simulink model "Power_Forcasting_V1_UseThisOne"  (R2024a)
settings: Solver=VariableStepAuto  StartTime=0.0  StopTime=2154  RelTol=1e-3
undefined symbols (not defined in the file or in its folder): DiscIntNeverNeededParam
libraries: dspstat3 x2, slpidlib x1
settings Model: Creator=ezeki  LastModifiedBy=ezeki

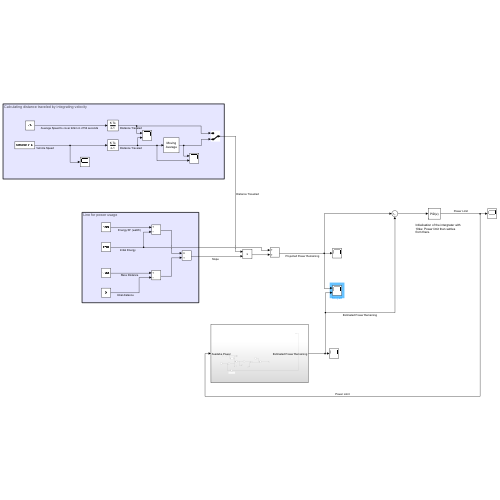
[thumbnail: Simulink's stored preview of the top-level diagram]
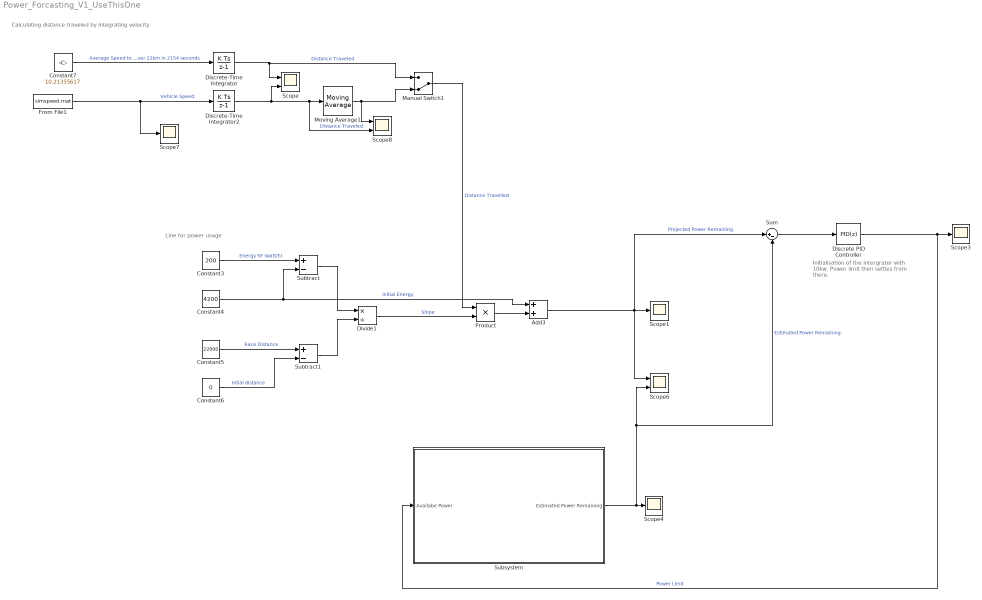
== system Power_Forcasting_V1_UseThisOne ==
  note: Calculating distance traveled by integrating velocity
  note: Line for power usage
  note: Initialisation of the intergrater with 10kw. Power limit then settles from there.
  Add3 : Sum
  Constant3 : Constant  Value=200
  Constant4 : Constant  Value=4200
  Constant5 : Constant  Value=22000
  Constant6 : Constant  Value=0
  Constant7 : Constant  Value=10.21355617
  Discrete PID Controller : slpidlib/PID Controller  Controller=PID  Form=Parallel  TimeDomain=Discrete-time  UseExternalTs=off  SampleTime=-1  IntegratorMethod=Forward Euler  FilterMethod=Forward Euler  ControllerParametersSource=internal  P=-10  I=0.001  UseKiTs=off  D=500  UseExternalDerivativeSource=off  N=0.01  UseFilter=on  TunerSelectOption=Transfer Function Based (PID Tuner App)  InitialConditionSource=internal  InitialConditionForIntegrator=10000  InitialConditionForFilter=0  DifferentiatorICPrevScaledInput=0  ExternalReset=none  TrackingMode=off  Kt=1  LimitOutput=off  SatLimitsSource=internal  UpperSaturationLimit=inf  LowerSaturationLimit=-inf  LinearizeAsGain=off  AntiWindupMode=none  Kb=1  LimitIntegrator=off  UpperIntegratorSaturationLimit=inf  LowerIntegratorSaturationLimit=-inf  POutMin=[]  POutMax=[]  IOutMin=[]  IOutMax=[]  DOutMin=[]  DOutMax=[]  NOutMin=[]  NOutMax=[]  SumOutMin=[]  SumOutMax=[]  SaturationOutMin=[]  SaturationOutMax=[]  PParamMin=[]  PParamMax=[]  IParamMin=[]  IParamMax=[]  DParamMin=[]  DParamMax=[]  NParamMin=[]  NParamMax=[]  KbParamMin=[]  KbParamMax=[]  KtParamMin=[]  KtParamMax=[]  KbOutMin=[]  KbOutMax=[]  KtOutMin=[]  KtOutMax=[]  IntegratorOutMin=[]  IntegratorOutMax=[]  FilterOutMin=[]  FilterOutMax=[]  SumI1OutMin=[]  SumI1OutMax=[]  SumI2OutMin=[]  SumI2OutMax=[]  SumI3OutMin=[]  SumI3OutMax=[]  SumI4OutMin=[]  SumI4OutMax=[]  SumDOutMin=[]  SumDOutMax=[]  DifferentiatorOutMin=[]  DifferentiatorOutMax=[]  FilterDiffOutCoefMin=[]  FilterDiffOutCoefMax=[]  ReciprocalOutMin=[]  ReciprocalOutMax=[]  SumDenOutMin=[]  SumDenOutMax=[]  SumNumOutMin=[]  SumNumOutMax=[]  DivideOutMin=[]  DivideOutMax=[]  UdiffTsProdOutMin=[]  UdiffTsProdOutMax=[]  NTsProdOutMin=[]  NTsProdOutMax=[]  UintegralTsProdOutMin=[]  UintegralTsProdOutMax=[]  UngainTsProdOutMin=[]  UngainTsProdOutMax=[]  ClampingZeroOutDataTypeStr=Inherit: Inherit via back propagation  ClampingZeroOutMin=[]  ClampingZeroOutMax=[]  FilterDenConstantOutDataTypeStr=Inherit: Inherit via back propagation  FilterDenConstantOutMin=[]  FilterDenConstantOutMax=[]  PCopyOutDataTypeStr=Inherit: Inherit via back propagation  PCopyOutMin=[]  PCopyOutMax=[]  NCopyOutDataTypeStr=Inherit: Inherit via back propagation  NCopyOutMin=[]  NCopyOutMax=[]  IntegratorContinuousStateAttributes=''  IntegratorStateMustResolveToSignalObject=off  IntegratorRTWStateStorageClass=Auto  FilterContinuousStateAttributes=''  FilterStateMustResolveToSignalObject=off  FilterRTWStateStorageClass=Auto  ParallelPVariant=InternalParameters  IdealPVariant=Disabled  IVariant=InternalParameters  DVariant=InternalParameters  IntegratorVariant=Discrete  SatVariant=Disabled  AWVariant=Passthrough  PCopyVariant=Disabled  TRVariant=Disabled  FdbkBlocksVariant=Forward  IdealPFdbkVariant=Disabled  SatFdbkVariant=Disabled  DerivativeFilterVariant=ForwardEulerFilter  NVariant=InternalParameters  NCopyVariant=Disabled  FilterICVariant=InternalICsFilter  IntegratorICVariant=InternalICs  ExternalResetVariant=Disabled  TRSumVariant=Passthrough  SumFdbkVariant=Disabled  SumVariant=Sum_PID  TsampFilterVariant=InternalTs  TsampNgainVariant=Passthrough  TsampIntegralVariant=Disabled_SignalSpec  ExternalSaturationOutDataTypeStr=Inherit: Same as second input  DerivativeSourceVariant=ErrorSignal
      settings: LibrarySourceBlock=simulink/Discrete/Discrete PID Controller
  Discrete-Time Integrator : DiscreteIntegrator  SampleTime=0.01  ICPrevOutput=DiscIntNeverNeededParam  ICPrevScaledInput=DiscIntNeverNeededParam
  Discrete-Time Integrator2 : DiscreteIntegrator  SampleTime=0.01  ICPrevOutput=DiscIntNeverNeededParam  ICPrevScaledInput=DiscIntNeverNeededParam
  Divide1 : Product  Inputs=*/
  From File1 : FromFile  FileName=simspeed.mat  SampleTime=0.01
  Manual Switch1 : ManualSwitch  CurrentSetting=0
  Moving Average1 : dspstat3/Moving Average  Method=Sliding window  ForgettingFactorPort=off  SpecifyWindowLength=on  WindowLength=1000  OverlapLength=999  AllowArbitraryInputLength=off  ForgettingFactor=0.9  SimulateUsing=Interpreted execution
  Product : Product
  Scope : Scope  NumInputPorts=2
  Scope{1,3..4,7} (4 alike) : Scope
  Scope6 : Scope  NumInputPorts=2
  Scope8 : Scope  NumInputPorts=2
  Subsystem : Subsystem
  Subtract : Sum  Inputs=+-
  Subtract1 : Sum  Inputs=+-
  Sum : Sum  Inputs=|+-
  wires:
  Discrete-Time Integrator/1 -> Manual Switch1/1, Scope/1  "Distance Traveled"
  Constant3/1 -> Subtract/1  "Energy SF (watt/h)"
  Constant4/1 -> Add3/1, Subtract/2  "Initial Energy"
  Constant6/1 -> Subtract1/2  "Intial distance"
  Constant5/1 -> Subtract1/1  "Race Distance"
  Subtract/1 -> Divide1/1
  Subtract1/1 -> Divide1/2
  Divide1/1 -> Product/2  "Slope"
  Product/1 -> Add3/2
  Add3/1 -> Scope6/1, Sum/1, Scope1/1  "Projected Power Remaining"
  Constant7/1 -> Discrete-Time Integrator/1  "Average Speed to cover 22km in 2154 seconds"
  Sum/1 -> Discrete PID Controller/1
  From File1/1 -> Scope7/1, Discrete-Time Integrator2/1  "Vehicle Speed"
  Discrete-Time Integrator2/1 -> Scope/2, Scope8/2, Moving Average1/1  "Distance Traveled"
  Discrete PID Controller/1 -> Subsystem/1(Availabe Power), Scope3/1  "Power Limit"
  Manual Switch1/1 -> Product/1  "Distance Travelled"
  Moving Average1/1 -> Scope8/1, Manual Switch1/2
  Subsystem/1(Estimated Power Remaining) -> Sum/2, Scope6/2, Scope4/1  "Estimated Power Remaining"

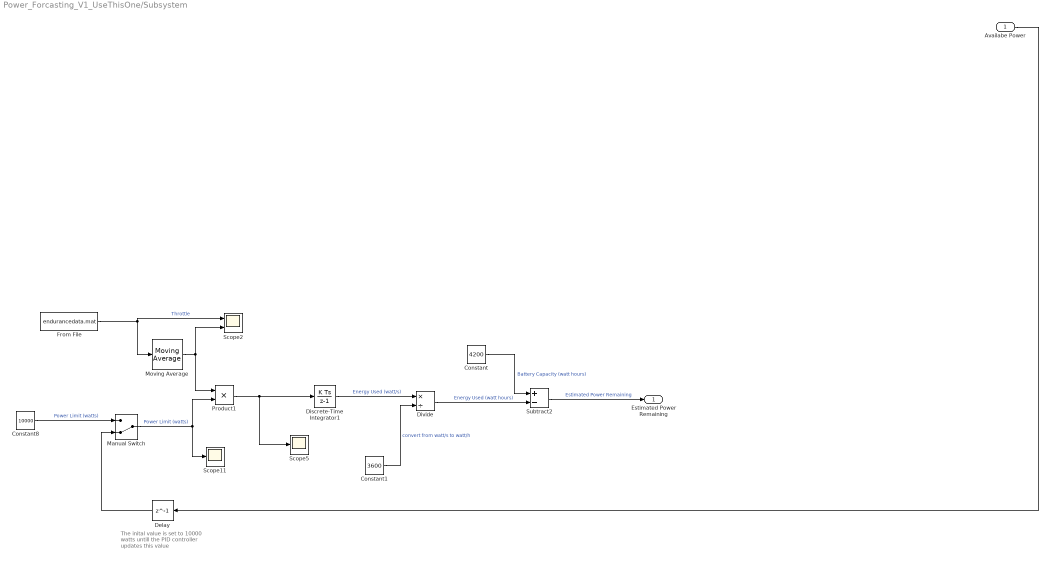
== system Power_Forcasting_V1_UseThisOne/Subsystem ==
  note: The inital value is set to 10000 watts untill the PID controller updates this value
  Availabe Power : Inport
  Constant : Constant  Value=4200
  Constant1 : Constant  Value=3600
  Constant8 : Constant  Value=10000
  Delay : Delay  DelayLength=1  InitialCondition=10000
  Discrete-Time Integrator1 : DiscreteIntegrator  SampleTime=0.01  ICPrevOutput=DiscIntNeverNeededParam  ICPrevScaledInput=DiscIntNeverNeededParam
  Divide : Product  Inputs=*/
  From File : FromFile  FileName=endurancedata.mat  SampleTime=0.01
  Manual Switch : ManualSwitch  CurrentSetting=0
  Moving Average : dspstat3/Moving Average  Method=Sliding window  ForgettingFactorPort=off  SpecifyWindowLength=on  WindowLength=1000  OverlapLength=999  AllowArbitraryInputLength=off  ForgettingFactor=0.9  SimulateUsing=Interpreted execution
  Product1 : Product
  Scope11 : Scope
  Scope2 : Scope  NumInputPorts=2
  Scope5 : Scope
  Subtract2 : Sum  Inputs=+-
  Estimated Power Remaining : Outport
  wires:
  From File/1 -> Scope2/1, Moving Average/1  "Throttle"
  Constant1/1 -> Divide/2  "convert from watt/s to watt/h"
  Divide/1 -> Subtract2/2  "Energy Used (watt hours)"
  Manual Switch/1 -> Scope11/1, Product1/2  "Power Limit (watts)"
  Moving Average/1 -> Scope2/2, Product1/1
  Constant/1 -> Subtract2/1  "Battery Capacity (watt hours)"
  Discrete-Time Integrator1/1 -> Divide/1  "Energy Used (watt/s)"
  Product1/1 -> Scope5/1, Discrete-Time Integrator1/1
  Availabe Power/1 -> Delay/1
  Constant8/1 -> Manual Switch/1  "Power Limit (watts)"
  Subtract2/1 -> Estimated Power Remaining/1  "Estimated Power Remaining"
  Delay/1 -> Manual Switch/2
